simulink model "npc_controller"  (R2022a)
settings: Solver=FixedStepDiscrete  StartTime=0.0  StopTime=20  RelTol=1e-3  EnableMultiTasking=on
values from neighbouring files (symbols this model uses):
  Tsw = 1.5E-5    [param.sldd]
undefined symbols (not defined in the file or in its folder): CAN_O_INT, CANA_BASE, Down, GPTRIP1SEL, GPTRIP2SEL, GPTRIP3SEL, TZ1, TZ2, TZ3, Up
libraries: simulink x153, hdlsllib x90, c2802xlib x34, c2837xDlib x18, c280xlib x12, canmsglib x9, c2838xlib x8, idelinklib_common x3, c2806xlib x2, slpidlib x2, c28004xlib x2, c281xlib x2
(part 38 of 45)

== system npc_controller/CONTROL/STATE-MACHINE/CPU_CONTROL_750_A2_precharge_pfc_ok2_OL SS2/updateSequencePhB/pol_vxn1/neg/SR ON ==
  note: Note:
      | AQCSFRC
      | 0b00 - disables forced PWM
      | 0b01 - forces PWM to LOW
      | 0b10 - forces PWM to  HIGH
  note: Note:A2
      |
      | Function PWM # GPIO # LAUNCHPAD PIN #
      |
      | Synci EPWM1A GPIO0 J4.40
      | EPWM1B GPIO1 J4.39
      |
      | ORPS EPMW6A GPIO10 J8.76
      | EPWM6B GPIO11 J8.75
      |
      | RELAY EPWM3A GPIO4 J4.36
      |
      | TZ GPIO62 XX
      |
      | a_s1 EPWM2A GPIO2 J4.38 XBAR_TRIP4
      | a_s2 EPWM7B GPIO13 XX
      | a_s3 EPWM2B GPIO3 J4.37
      | a_s4 EPWM7A GPIO12 XX XBAR_TRIP5
      |
      | b_s1 EPWM8B GPIO15 J8.73 XBAR_TRIP7
      | b_s2 EPWM9B GPIO17 XX
      | b_s3 EPWM8A GPIO14 J8.74
      | b_s4 EPWM9A GPIO16 J4.33 XBAR_TRIP8
      |
      | c_s1 EPWM10B GPIO19 J1.3 XBAR_TRIP9
      | c_s2 EPWM11B GPIO21 XX
      | c_s3 EPWM10A GPIO18 J1.4
      | c_s4 EPWM11A GPIO20 XX XBAR_TRIP10
  note: EPwm8Regs.AQCSFRC.bit.CSFB = (uint16_T)(0b01);
      | EPwm9Regs.AQCSFRC.bit.CSFB = (uint16_T)(0b00);
      | EPwm8Regs.AQCSFRC.bit.CSFA = (uint16_T)(0b10);
      | EPwm9Regs.AQCSFRC.bit.CSFA = (uint16_T)(0b00);
  Action Port : ActionPort  ActionPortLabel=else
  Constant : Constant  Value=2  OutDataTypeStr=uint8  SampleTime=-1
  System Outputs1 : Subsystem  mask(System Outputs){ShowInLibBrowser=0}
      mask prompts: ShowInLibBrowser "Simulink:masks:CustCodeMaskParam1_MP"
      settings: CopyFcn=cccopyfcn(gcb)  OpenFcn=ccopenfcn('System Outputs Function')
      mask Help: eval('feval(''rtwprivate'',''rtwhelpview'',''rtw_sys_outputs_block'')');
      mask Display: disp('System\nOutputs');
  Out1 : Outport
  wires:
  Constant/1 -> Out1/1

== system npc_controller/CONTROL/STATE-MACHINE/CPU_CONTROL_750_A2_precharge_pfc_ok2_OL SS2/updateSequencePhB/pol_vxn1/pos/SR Force to Low ==
  note: Note:A2
      |
      | Function PWM # GPIO # LAUNCHPAD PIN #
      |
      | Synci EPWM1A GPIO0 J4.40
      | EPWM1B GPIO1 J4.39
      |
      | ORPS EPMW6A GPIO10 J8.76
      | EPWM6B GPIO11 J8.75
      |
      | RELAY EPWM3A GPIO4 J4.36
      |
      | TZ GPIO62 XX
      |
      | a_s1 EPWM2A GPIO2 J4.38 XBAR_TRIP4
      | a_s2 EPWM7B GPIO13 XX
      | a_s3 EPWM2B GPIO3 J4.37
      | a_s4 EPWM7A GPIO12 XX XBAR_TRIP5
      |
      | b_s1 EPWM8B GPIO15 J8.73 XBAR_TRIP7
      | b_s2 EPWM9B GPIO17 XX
      | b_s3 EPWM8A GPIO14 J8.74
      | b_s4 EPWM9A GPIO16 J4.33 XBAR_TRIP8
      |
      | c_s1 EPWM10B GPIO19 J1.3 XBAR_TRIP9
      | c_s2 EPWM11B GPIO21 XX
      | c_s3 EPWM10A GPIO18 J1.4
      | c_s4 EPWM11A GPIO20 XX XBAR_TRIP10
  note: Note:
      | AQCSFRC
      | 0b00 - disables forced PWM
      | 0b01 - forces PWM to LOW
      | 0b10 - forces PWM to  HIGH
  note: EPwm8Regs.AQCSFRC.bit.CSFB = (uint16_T)(0b01);
      | EPwm9Regs.AQCSFRC.bit.CSFB = (uint16_T)(0b10);
      | EPwm8Regs.AQCSFRC.bit.CSFA = (uint16_T)(0b00);
      | EPwm9Regs.AQCSFRC.bit.CSFA = (uint16_T)(0b01);
  Action Port : ActionPort  ActionPortLabel="if((u1 > -48)  & (u1 < 48))"
  Constant : Constant  OutDataTypeStr=uint8  SampleTime=-1
  System Outputs2 : Subsystem  mask(System Outputs){ShowInLibBrowser=0}
      mask prompts: ShowInLibBrowser "Simulink:masks:CustCodeMaskParam1_MP"
      settings: CopyFcn=cccopyfcn(gcb)  OpenFcn=ccopenfcn('System Outputs Function')
      mask Help: eval('feval(''rtwprivate'',''rtwhelpview'',''rtw_sys_outputs_block'')');
      mask Display: disp('System\nOutputs');
  Out1 : Outport
  wires:
  Constant/1 -> Out1/1

== system npc_controller/CONTROL/STATE-MACHINE/CPU_CONTROL_750_A2_precharge_pfc_ok2_OL SS2/updateSequencePhB/pol_vxn1/pos/SR ON ==
  note: Note:
      | AQCSFRC
      | 0b00 - disables forced PWM/pass through
      | 0b01 - forces PWM to LOW
      | 0b10 - forces PWM to  HIGH
  note: Note:A2
      |
      | Function PWM # GPIO # LAUNCHPAD PIN #
      |
      | Synci EPWM1A GPIO0 J4.40
      | EPWM1B GPIO1 J4.39
      |
      | ORPS EPMW6A GPIO10 J8.76
      | EPWM6B GPIO11 J8.75
      |
      | RELAY EPWM3A GPIO4 J4.36
      |
      | TZ GPIO62 XX
      |
      | a_s1 EPWM2A GPIO2 J4.38 XBAR_TRIP4
      | a_s2 EPWM7B GPIO13 XX
      | a_s3 EPWM2B GPIO3 J4.37
      | a_s4 EPWM7A GPIO12 XX XBAR_TRIP5
      |
      | b_s1 EPWM8B GPIO15 J8.73 XBAR_TRIP7
      | b_s2 EPWM9B GPIO17 XX
      | b_s3 EPWM8A GPIO14 J8.74
      | b_s4 EPWM9A GPIO16 J4.33 XBAR_TRIP8
      |
      | c_s1 EPWM10B GPIO19 J1.3 XBAR_TRIP9
      | c_s2 EPWM11B GPIO21 XX
      | c_s3 EPWM10A GPIO18 J1.4
      | c_s4 EPWM11A GPIO20 XX XBAR_TRIP10
  note: EPwm8Regs.AQCSFRC.bit.CSFB = (uint16_T)(0b00);
      | EPwm9Regs.AQCSFRC.bit.CSFB = (uint16_T)(0b10);
      | EPwm8Regs.AQCSFRC.bit.CSFA = (uint16_T)(0b00);
      | EPwm9Regs.AQCSFRC.bit.CSFA = (uint16_T)(0b01);
  Action Port : ActionPort  ActionPortLabel=else
  Constant : Constant  OutDataTypeStr=uint8  SampleTime=-1
  System Outputs1 : Subsystem  mask(System Outputs){ShowInLibBrowser=0}
      mask prompts: ShowInLibBrowser "Simulink:masks:CustCodeMaskParam1_MP"
      settings: CopyFcn=cccopyfcn(gcb)  OpenFcn=ccopenfcn('System Outputs Function')
      mask Help: eval('feval(''rtwprivate'',''rtwhelpview'',''rtw_sys_outputs_block'')');
      mask Display: disp('System\nOutputs');
  Out1 : Outport
  wires:
  Constant/1 -> Out1/1

== system npc_controller/CONTROL/STATE-MACHINE/CPU_CONTROL_750_A2_precharge_pfc_ok2_OL SS2/updateSequencePhB/pol_vxn1/zero/System Outputs1 ==

== system npc_controller/CONTROL/STATE-MACHINE/CPU_CONTROL_750_A2_precharge_pfc_ok2_OL SS2/updateSequencePhB/pol_vxn2/neg/System Outputs1 ==

== system npc_controller/CONTROL/STATE-MACHINE/CPU_CONTROL_750_A2_precharge_pfc_ok2_OL SS2/updateSequencePhB/pol_vxn2/neg/System Outputs2 ==

== system npc_controller/CONTROL/STATE-MACHINE/CPU_CONTROL_750_A2_precharge_pfc_ok2_OL SS2/updateSequencePhB/pol_vxn2/pos/System Outputs1 ==

== system npc_controller/CONTROL/STATE-MACHINE/CPU_CONTROL_750_A2_precharge_pfc_ok2_OL SS2/updateSequencePhB/pol_vxn2/pos/System Outputs2 ==

== system npc_controller/CONTROL/STATE-MACHINE/CPU_CONTROL_750_A2_precharge_pfc_ok2_OL SS2/updateSequencePhB/pol_vxn2/zero/System Outputs1 ==

== system npc_controller/CONTROL/STATE-MACHINE/CPU_CONTROL_750_A2_precharge_pfc_ok2_OL SS2/updateSequencePhC/pol_final1/prot/System Outputs ==

== system npc_controller/CONTROL/STATE-MACHINE/CPU_CONTROL_750_A2_precharge_pfc_ok2_OL SS2/updateSequencePhC/pol_vxn1/neg/SR OFF ==
  note: Note:A2
      |
      | Function PWM # GPIO # LAUNCHPAD PIN #
      |
      | Synci EPWM1A GPIO0 J4.40
      | EPWM1B GPIO1 J4.39
      |
      | ORPS EPMW6A GPIO10 J8.76
      | EPWM6B GPIO11 J8.75
      |
      | RELAY EPWM3A GPIO4 J4.36
      |
      | TZ GPIO62 XX
      |
      | a_s1 EPWM2A GPIO2 J4.38 XBAR_TRIP4
      | a_s2 EPWM7B GPIO13 XX
      | a_s3 EPWM2B GPIO3 J4.37
      | a_s4 EPWM7A GPIO12 XX XBAR_TRIP5
      |
      | b_s1 EPWM8B GPIO15 J8.73 XBAR_TRIP7
      | b_s2 EPWM9B GPIO17 XX
      | b_s3 EPWM8A GPIO14 J8.74
      | b_s4 EPWM9A GPIO16 J4.33 XBAR_TRIP8
      |
      | c_s1 EPWM10B GPIO19 J1.3 XBAR_TRIP9
      | c_s2 EPWM11B GPIO21 XX
      | c_s3 EPWM10A GPIO18 J1.4
      | c_s4 EPWM11A GPIO20 XX XBAR_TRIP10
  note: Note:
      | AQCSFRC
      | 0b00 - disables forced PWM
      | 0b01 - forces PWM to LOW
      | 0b10 - forces PWM to  HIGH
  note: EPwm10Regs.AQCSFRC.bit.CSFB = (uint16_T)(0b01);
      | EPwm11Regs.AQCSFRC.bit.CSFB = (uint16_T)(0b00);
      | EPwm10Regs.AQCSFRC.bit.CSFA = (uint16_T)(0b10);
      | EPwm11Regs.AQCSFRC.bit.CSFA = (uint16_T)(0b01);
  Action Port : ActionPort  ActionPortLabel="if((u1 > -48)  & (u1 < 48))"
  Constant : Constant  Value=2  OutDataTypeStr=uint8  SampleTime=-1
  System Outputs1 : Subsystem  mask(System Outputs){ShowInLibBrowser=0}
      mask prompts: ShowInLibBrowser "Simulink:masks:CustCodeMaskParam1_MP"
      settings: CopyFcn=cccopyfcn(gcb)  OpenFcn=ccopenfcn('System Outputs Function')
      mask Help: eval('feval(''rtwprivate'',''rtwhelpview'',''rtw_sys_outputs_block'')');
      mask Display: disp('System\nOutputs');
  Out1 : Outport
  wires:
  Constant/1 -> Out1/1

== system npc_controller/CONTROL/STATE-MACHINE/CPU_CONTROL_750_A2_precharge_pfc_ok2_OL SS2/updateSequencePhC/pol_vxn1/neg/SR ON ==
  note: Note:
      | AQCSFRC
      | 0b00 - disables forced PWM
      | 0b01 - forces PWM to LOW
      | 0b10 - forces PWM to  HIGH
  note: Note:A2
      |
      | Function PWM # GPIO # LAUNCHPAD PIN #
      |
      | Synci EPWM1A GPIO0 J4.40
      | EPWM1B GPIO1 J4.39
      |
      | ORPS EPMW6A GPIO10 J8.76
      | EPWM6B GPIO11 J8.75
      |
      | RELAY EPWM3A GPIO4 J4.36
      |
      | TZ GPIO62 XX
      |
      | a_s1 EPWM2A GPIO2 J4.38 XBAR_TRIP4
      | a_s2 EPWM7B GPIO13 XX
      | a_s3 EPWM2B GPIO3 J4.37
      | a_s4 EPWM7A GPIO12 XX XBAR_TRIP5
      |
      | b_s1 EPWM8B GPIO15 J8.73 XBAR_TRIP7
      | b_s2 EPWM9B GPIO17 XX
      | b_s3 EPWM8A GPIO14 J8.74
      | b_s4 EPWM9A GPIO16 J4.33 XBAR_TRIP8
      |
      | c_s1 EPWM10B GPIO19 J1.3 XBAR_TRIP9
      | c_s2 EPWM11B GPIO21 XX
      | c_s3 EPWM10A GPIO18 J1.4
      | c_s4 EPWM11A GPIO20 XX XBAR_TRIP10
  note: EPwm10Regs.AQCSFRC.bit.CSFB = (uint16_T)(0b01);
      | EPwm11Regs.AQCSFRC.bit.CSFB = (uint16_T)(0b00);
      | EPwm10Regs.AQCSFRC.bit.CSFA = (uint16_T)(0b10);
      | EPwm11Regs.AQCSFRC.bit.CSFA = (uint16_T)(0b00);
  Action Port : ActionPort  ActionPortLabel=else
  Constant : Constant  Value=2  OutDataTypeStr=uint8  SampleTime=-1
  System Outputs1 : Subsystem  mask(System Outputs){ShowInLibBrowser=0}
      mask prompts: ShowInLibBrowser "Simulink:masks:CustCodeMaskParam1_MP"
      settings: CopyFcn=cccopyfcn(gcb)  OpenFcn=ccopenfcn('System Outputs Function')
      mask Help: eval('feval(''rtwprivate'',''rtwhelpview'',''rtw_sys_outputs_block'')');
      mask Display: disp('System\nOutputs');
  Out1 : Outport
  wires:
  Constant/1 -> Out1/1

== system npc_controller/CONTROL/STATE-MACHINE/CPU_CONTROL_750_A2_precharge_pfc_ok2_OL SS2/updateSequencePhC/pol_vxn1/pos/SR Force to Low ==
  note: Note:A2
      |
      | Function PWM # GPIO # LAUNCHPAD PIN #
      |
      | Synci EPWM1A GPIO0 J4.40
      | EPWM1B GPIO1 J4.39
      |
      | ORPS EPMW6A GPIO10 J8.76
      | EPWM6B GPIO11 J8.75
      |
      | RELAY EPWM3A GPIO4 J4.36
      |
      | TZ GPIO62 XX
      |
      | a_s1 EPWM2A GPIO2 J4.38 XBAR_TRIP4
      | a_s2 EPWM7B GPIO13 XX
      | a_s3 EPWM2B GPIO3 J4.37
      | a_s4 EPWM7A GPIO12 XX XBAR_TRIP5
      |
      | b_s1 EPWM8B GPIO15 J8.73 XBAR_TRIP7
      | b_s2 EPWM9B GPIO17 XX
      | b_s3 EPWM8A GPIO14 J8.74
      | b_s4 EPWM9A GPIO16 J4.33 XBAR_TRIP8
      |
      | c_s1 EPWM10B GPIO19 J1.3 XBAR_TRIP9
      | c_s2 EPWM11B GPIO21 XX
      | c_s3 EPWM10A GPIO18 J1.4
      | c_s4 EPWM11A GPIO20 XX XBAR_TRIP10
  note: Note:
      | AQCSFRC
      | 0b00 - disables forced PWM
      | 0b01 - forces PWM to LOW
      | 0b10 - forces PWM to  HIGH
  note: EPwm10Regs.AQCSFRC.bit.CSFB = (uint16_T)(0b01);
      | EPwm11Regs.AQCSFRC.bit.CSFB = (uint16_T)(0b10);
      | EPwm10Regs.AQCSFRC.bit.CSFA = (uint16_T)(0b00);
      | EPwm11Regs.AQCSFRC.bit.CSFA = (uint16_T)(0b01);
  Action Port : ActionPort  ActionPortLabel="if((u1 > -48)  & (u1 < 48))"
  Constant : Constant  OutDataTypeStr=uint8  SampleTime=-1
  System Outputs2 : Subsystem  mask(System Outputs){ShowInLibBrowser=0}
      mask prompts: ShowInLibBrowser "Simulink:masks:CustCodeMaskParam1_MP"
      settings: CopyFcn=cccopyfcn(gcb)  OpenFcn=ccopenfcn('System Outputs Function')
      mask Help: eval('feval(''rtwprivate'',''rtwhelpview'',''rtw_sys_outputs_block'')');
      mask Display: disp('System\nOutputs');
  Out1 : Outport
  wires:
  Constant/1 -> Out1/1

== system npc_controller/CONTROL/STATE-MACHINE/CPU_CONTROL_750_A2_precharge_pfc_ok2_OL SS2/updateSequencePhC/pol_vxn1/pos/SR ON ==
  note: Note:
      | AQCSFRC
      | 0b00 - disables forced PWM/pass through
      | 0b01 - forces PWM to LOW
      | 0b10 - forces PWM to  HIGH
  note: Note:A2
      |
      | Function PWM # GPIO # LAUNCHPAD PIN #
      |
      | Synci EPWM1A GPIO0 J4.40
      | EPWM1B GPIO1 J4.39
      |
      | ORPS EPMW6A GPIO10 J8.76
      | EPWM6B GPIO11 J8.75
      |
      | RELAY EPWM3A GPIO4 J4.36
      |
      | TZ GPIO62 XX
      |
      | a_s1 EPWM2A GPIO2 J4.38 XBAR_TRIP4
      | a_s2 EPWM7B GPIO13 XX
      | a_s3 EPWM2B GPIO3 J4.37
      | a_s4 EPWM7A GPIO12 XX XBAR_TRIP5
      |
      | b_s1 EPWM8B GPIO15 J8.73 XBAR_TRIP7
      | b_s2 EPWM9B GPIO17 XX
      | b_s3 EPWM8A GPIO14 J8.74
      | b_s4 EPWM9A GPIO16 J4.33 XBAR_TRIP8
      |
      | c_s1 EPWM10B GPIO19 J1.3 XBAR_TRIP9
      | c_s2 EPWM11B GPIO21 XX
      | c_s3 EPWM10A GPIO18 J1.4
      | c_s4 EPWM11A GPIO20 XX XBAR_TRIP10
  note: EPwm10Regs.AQCSFRC.bit.CSFB = (uint16_T)(0b00);
      | EPwm11Regs.AQCSFRC.bit.CSFB = (uint16_T)(0b10);
      | EPwm10Regs.AQCSFRC.bit.CSFA = (uint16_T)(0b00);
      | EPwm11Regs.AQCSFRC.bit.CSFA = (uint16_T)(0b01);
  Action Port : ActionPort  ActionPortLabel=else
  Constant : Constant  OutDataTypeStr=uint8  SampleTime=-1
  System Outputs1 : Subsystem  mask(System Outputs){ShowInLibBrowser=0}
      mask prompts: ShowInLibBrowser "Simulink:masks:CustCodeMaskParam1_MP"
      settings: CopyFcn=cccopyfcn(gcb)  OpenFcn=ccopenfcn('System Outputs Function')
      mask Help: eval('feval(''rtwprivate'',''rtwhelpview'',''rtw_sys_outputs_block'')');
      mask Display: disp('System\nOutputs');
  Out1 : Outport
  wires:
  Constant/1 -> Out1/1

== system npc_controller/CONTROL/STATE-MACHINE/CPU_CONTROL_750_A2_precharge_pfc_ok2_OL SS2/updateSequencePhC/pol_vxn1/zero/System Outputs1 ==

== system npc_controller/CONTROL/STATE-MACHINE/CPU_CONTROL_750_A2_precharge_pfc_ok2_OL SS2/updateSequencePhC/pol_vxn2/neg/System Outputs1 ==

== system npc_controller/CONTROL/STATE-MACHINE/CPU_CONTROL_750_A2_precharge_pfc_ok2_OL SS2/updateSequencePhC/pol_vxn2/pos/System Outputs1 ==

== system npc_controller/CONTROL/STATE-MACHINE/CPU_CONTROL_750_A2_precharge_pfc_ok2_OL SS2/updateSequencePhC/pol_vxn2/pos/System Outputs2 ==

== system npc_controller/CONTROL/STATE-MACHINE/CPU_CONTROL_750_A2_precharge_pfc_ok2_OL SS2/updateSequencePhC/pol_vxn2/zero/System Outputs1 ==

== system npc_controller/CONTROL/STATE-MACHINE/CPU_CONTROL_750_Vpk/configGrid/FORCE_TZ/1P/ALL_LEGS ==
  note: Note:
      | TZCCTL
      | 0b00 - High impedance
      | 0b01 - Force to HIGH
      | 0b10 - Force to LOW
      | 0b11 - Do nothing
      |
      | AQCSFRC
      | 0b00 - disables forced PWM
      | 0b01 - forces PWM to LOW
      | 0b10 - forces PWM to  HIGH
      |
      | TZFRC.bit.OST
      | 0b0 - Do nothing
      | 0b1 - Force TZ
  note: EALLOW;
      |
      | /*Force TZ*/
      | EPwm6Regs. TZFRC.bit.OST = 0b0; //do nothing
      | EPwm7Regs. TZFRC.bit.OST = 0b0;
      | EPwm8Regs. TZFRC.bit.OST = 0b0;
      | EPwm9Regs. TZFRC.bit.OST = 0b0;
      | EPwm10Regs. TZFRC.bit.OST = 0b0;
      | EPwm11Regs. TZFRC.bit.OST = 0b0;
      |
      | EDIS;
      |
      | //change ref for leg B and legC
  Action Port : ActionPort
  System Outputs2 : Subsystem  mask(System Outputs){ShowInLibBrowser=0}
      mask prompts: ShowInLibBrowser "Simulink:masks:CustCodeMaskParam1_MP"
      settings: CopyFcn=cccopyfcn(gcb)  OpenFcn=ccopenfcn('System Outputs Function')
      mask Help: eval('feval(''rtwprivate'',''rtwhelpview'',''rtw_sys_outputs_block'')');
      mask Display: disp('System\nOutputs');

== system npc_controller/CONTROL/STATE-MACHINE/CPU_CONTROL_750_Vpk/configGrid/FORCE_TZ/1P/LEG_A ==
  note: EALLOW;
      |
      | /*Force TZ*/
      | EPwm6Regs. TZFRC.bit.OST = 0b0; //do nothing
      | EPwm7Regs. TZFRC.bit.OST = 0b0;
      | EPwm8Regs. TZFRC.bit.OST = 0b1;
      | EPwm9Regs. TZFRC.bit.OST = 0b1;
      | EPwm10Regs. TZFRC.bit.OST = 0b1;
      | EPwm11Regs. TZFRC.bit.OST = 0b1;
      |
      | EDIS;
  note: Note:
      | TZCCTL
      | 0b00 - High impedance
      | 0b01 - Force to HIGH
      | 0b10 - Force to LOW
      | 0b11 - Do nothing
      |
      | AQCSFRC
      | 0b00 - disables forced PWM
      | 0b01 - forces PWM to LOW
      | 0b10 - forces PWM to  HIGH
      |
      | TZFRC.bit.OST
      | 0b0 - Do nothing
      | 0b1 - Force TZ
  Action Port : ActionPort
  System Outputs2 : Subsystem  mask(System Outputs){ShowInLibBrowser=0}
      mask prompts: ShowInLibBrowser "Simulink:masks:CustCodeMaskParam1_MP"
      settings: CopyFcn=cccopyfcn(gcb)  OpenFcn=ccopenfcn('System Outputs Function')
      mask Help: eval('feval(''rtwprivate'',''rtwhelpview'',''rtw_sys_outputs_block'')');
      mask Display: disp('System\nOutputs');

== system npc_controller/CONTROL/STATE-MACHINE/CPU_CONTROL_750_Vpk/configGrid/FORCE_TZ/1P/LEG_B ==
  note: Note:
      | TZCCTL
      | 0b00 - High impedance
      | 0b01 - Force to HIGH
      | 0b10 - Force to LOW
      | 0b11 - Do nothing
      |
      | AQCSFRC
      | 0b00 - disables forced PWM
      | 0b01 - forces PWM to LOW
      | 0b10 - forces PWM to  HIGH
      |
      | TZFRC.bit.OST
      | 0b0 - Do nothing
      | 0b1 - Force TZ
  note: EALLOW;
      |
      | /*Force TZ*/
      | EPwm6Regs. TZFRC.bit.OST = 0b1; //do nothing
      | EPwm7Regs. TZFRC.bit.OST = 0b1;
      | EPwm8Regs. TZFRC.bit.OST = 0b0;
      | EPwm9Regs. TZFRC.bit.OST = 0b0;
      | EPwm10Regs. TZFRC.bit.OST = 0b1;
      | EPwm11Regs. TZFRC.bit.OST = 0b1;
      |
      | EDIS;
  Action Port : ActionPort
  System Outputs2 : Subsystem  mask(System Outputs){ShowInLibBrowser=0}
      mask prompts: ShowInLibBrowser "Simulink:masks:CustCodeMaskParam1_MP"
      settings: CopyFcn=cccopyfcn(gcb)  OpenFcn=ccopenfcn('System Outputs Function')
      mask Help: eval('feval(''rtwprivate'',''rtwhelpview'',''rtw_sys_outputs_block'')');
      mask Display: disp('System\nOutputs');

== system npc_controller/CONTROL/STATE-MACHINE/CPU_CONTROL_750_Vpk/configGrid/FORCE_TZ/1P/LEG_C ==
  note: EALLOW;
      |
      | /*Force TZ*/
      | EPwm6Regs. TZFRC.bit.OST = 0b1; //do nothing
      | EPwm7Regs. TZFRC.bit.OST = 0b1;
      | EPwm8Regs. TZFRC.bit.OST = 0b1;
      | EPwm9Regs. TZFRC.bit.OST = 0b1;
      | EPwm10Regs. TZFRC.bit.OST = 0b0;
      | EPwm11Regs. TZFRC.bit.OST = 0b0;
      |
      | EDIS;
  note: Note:
      | TZCCTL
      | 0b00 - High impedance
      | 0b01 - Force to HIGH
      | 0b10 - Force to LOW
      | 0b11 - Do nothing
      |
      | AQCSFRC
      | 0b00 - disables forced PWM
      | 0b01 - forces PWM to LOW
      | 0b10 - forces PWM to  HIGH
      |
      | TZFRC.bit.OST
      | 0b0 - Do nothing
      | 0b1 - Force TZ
  Action Port : ActionPort
  System Outputs2 : Subsystem  mask(System Outputs){ShowInLibBrowser=0}
      mask prompts: ShowInLibBrowser "Simulink:masks:CustCodeMaskParam1_MP"
      settings: CopyFcn=cccopyfcn(gcb)  OpenFcn=ccopenfcn('System Outputs Function')
      mask Help: eval('feval(''rtwprivate'',''rtwhelpview'',''rtw_sys_outputs_block'')');
      mask Display: disp('System\nOutputs');

== system npc_controller/CONTROL/STATE-MACHINE/CPU_CONTROL_750_Vpk/configGrid/FORCE_TZ/3P3W/System Outputs2 ==

== system npc_controller/CONTROL/STATE-MACHINE/CPU_CONTROL_750_Vpk/updateCalib/done/RESET_TZ/System Outputs2 ==

== system npc_controller/CONTROL/STATE-MACHINE/CPU_CONTROL_750_Vpk/updatePll3p/PLL/SRF_PLL/Integrator ==
  PI Out : Inport  OutDataTypeStr=single
  Accumulation : Subsystem  TreatAsAtomicUnit=on
  Add : Sum  AccumDataTypeStr=single
  Compare To Constant : simulink/Logic and Bit Operations/Compare To Constant  relop=>=  const=2*pi  OutDataTypeStr=boolean
  If : If  IfExpression=u1
  Merge : Merge
  Product : Product  OutDataTypeStr=single
  Reset Integrator : Subsystem  TreatAsAtomicUnit=on
  Ts : Constant  Value=Tsw  OutDataTypeStr=single
  Unit Delay : UnitDelay  SampleTime=-1  HasFrameUpgradeWarning=on
  wt : Outport
  wires:
  PI Out/1 -> Product/1
  Ts/1 -> Product/2
  Product/1 -> Add/1
  Add/1 -> Accumulation/1(In1), Compare To Constant/1
  Compare To Constant/1 -> If/1
  If/1 -> Reset Integrator/Action
  If/2 -> Accumulation/Action
  Reset Integrator/1(Out) -> Merge/1
  Accumulation/1(Out) -> Merge/2
  Merge/1 -> Unit Delay/1
  Unit Delay/1 -> wt/1, Add/2

== system npc_controller/CONTROL/STATE-MACHINE/CPU_CONTROL_750_Vpk/updatePll3p/PLL/SRF_PLL/PI ==
  Vq : Inport
  Ki : Gain  Gain=200
  Ki1 : Gain  Commented=on  Gain=200
  Kp : Gain  Gain=0.5
  Kp1 : Gain  Commented=on  Gain=0.5
  Sum : Sum  Inputs=|++
  Sum1 : Sum  Inputs=+|+
  Ts/2 : Gain  Gain=Tsw/2
  Unit Delay : UnitDelay  SampleTime=-1  HasFrameUpgradeWarning=on
  PI Out : Outport
  wires:
  Ts/2/1 -> Sum/1
  Sum1/1 -> PI Out/1
  Ki/1 -> Ts/2/1
  Vq/1 -> Ki/1, Kp/1  "Vq"
  Unit Delay/1 -> Sum/2
  Kp/1 -> Sum1/1
  Sum/1 -> Sum1/2, Unit Delay/1

== system npc_controller/CONTROL/STATE-MACHINE/CPU_CONTROL_750_Vpk/updatePll3p/PLL/SRF_PLL/Subsystem1 ==
  x[n] : Inport
  1 - Lambda : Gain  Gain=1 - 0.98
  Delay : Delay  DelayLength=1
  Gain{,1..7} (8 alike) : Gain  Commented=on  Gain=1/8
  Lambda : Gain  Gain=0.98
  Memory{,1..6} (7 alike) : Memory  Commented=on  InheritSampleTime=on
  Sum{,1..6} (7 alike) : Sum  Commented=on  Inputs=++|
  Sum7 : Sum  Inputs=|++
  y[n] : Outport
  wires:
  Sum7/1 -> y[n]/1, Delay/1
  Delay/1 -> Lambda/1
  1 - Lambda/1 -> Sum7/1
  x[n]/1 -> 1 - Lambda/1
  Lambda/1 -> Sum7/2
  Gain7/1 -> Sum6/1
  Sum5/1 -> Sum6/2
  Memory6/1 -> Gain7/1
  Memory5/1 -> Gain6/1, Memory6/1
  Sum4/1 -> Sum5/2
  Gain6/1 -> Sum5/1
  Gain5/1 -> Sum4/1
  Sum3/1 -> Sum4/2
  Memory4/1 -> Gain5/1, Memory5/1
  Memory3/1 -> Gain4/1, Memory4/1
  Sum2/1 -> Sum3/2
  Gain4/1 -> Sum3/1
  Gain3/1 -> Sum2/1
  Sum1/1 -> Sum2/2
  Gain2/1 -> Sum1/1
  Sum/1 -> Sum1/2
  Gain1/1 -> Sum/1
  Gain/1 -> Sum/2
  Memory2/1 -> Gain3/1, Memory3/1
  Memory1/1 -> Gain2/1, Memory2/1
  Memory/1 -> Gain1/1, Memory1/1

== system npc_controller/CONTROL/STATE-MACHINE/CPU_CONTROL_750_Vpk/updatePll3p/PLL/SRF_PLL/abc to dq ==
  note: wt
  note: wt
  note: wt
  a : Inport
  b : Inport  Port=2
  c : Inport  Port=3
  wt : Inport  Port=4
  (wt+120) : Sum  Inputs=|++
  (wt-120) : Sum  Inputs=|+-
  2pi_3 : Constant  Value=2*pi/3
  Add3 : Sum  Inputs=+++
  Cos3 : Trigonometry  Operator=cos
  Cos4 : Trigonometry  Operator=cos
  Cos5 : Trigonometry  Operator=cos
  Product5 : Product
  Product6 : Product
  Product7 : Product
  q1 : Gain  Gain=2/3
  q : Outport
  wires:
  [a] -> Product5/1
  Cos3/1 -> Product5/2
  wt/1 -> (wt+120)/1, (wt-120)/1, Cos3/1
  [ph] -> (wt+120)/2
  Product7/1 -> Add3/3
  a/1 -> [a]
  (wt+120)/1 -> Cos5/1
  Product6/1 -> Add3/2
  c/1 -> [c]
  [ph] -> (wt-120)/2
  (wt-120)/1 -> Cos4/1
  [b] -> Product6/1
  Cos4/1 -> Product6/2
  Product5/1 -> Add3/1
  Cos5/1 -> Product7/2
  b/1 -> [b]
  Add3/1 -> q1/1
  [c] -> Product7/1
  q1/1 -> q/1
  2pi_3/1 -> [ph]

== system npc_controller/CONTROL/STATE-MACHINE/CPU_CONTROL_750_Vpk/updatePll3p/PLL/Subsystem/Initialize at Zero Crossing ==
  In1 : Inport
  Trigger : TriggerPort  VariantControl=Variant
  OR : Logic  Operator=OR  IconShape=distinctive  AllPortsSameDT=off  OutDataTypeStr=boolean
  Unit Delay : UnitDelay  SampleTime=-1  HasFrameUpgradeWarning=on
  Out1 : Outport  InitialOutput=0  VectorParamsAs1DForOutWhenUnconnected=off
  wires:
  OR/1 -> Out1/1, Unit Delay/1
  Unit Delay/1 -> OR/2
  In1/1 -> OR/1

== system npc_controller/CONTROL/STATE-MACHINE/CPU_CONTROL_750_Vpk/updateSequencePhA/pol_final1/prot/System Outputs ==

== system npc_controller/CONTROL/STATE-MACHINE/CPU_CONTROL_750_Vpk/updateSequencePhA/pol_vxn1/neg/System Outputs1 ==

== system npc_controller/CONTROL/STATE-MACHINE/CPU_CONTROL_750_Vpk/updateSequencePhA/pol_vxn1/pos/System Outputs1 ==

== system npc_controller/CONTROL/STATE-MACHINE/CPU_CONTROL_750_Vpk/updateSequencePhA/pol_vxn1/pos/System Outputs2 ==

== system npc_controller/CONTROL/STATE-MACHINE/CPU_CONTROL_750_Vpk/updateSequencePhA/pol_vxn1/zero/System Outputs1 ==

== system npc_controller/CONTROL/STATE-MACHINE/CPU_CONTROL_750_Vpk/updateSequencePhB/pol_final1/prot/System Outputs ==

== system npc_controller/CONTROL/STATE-MACHINE/CPU_CONTROL_750_Vpk/updateSequencePhB/pol_vxn1/neg/System Outputs1 ==

== system npc_controller/CONTROL/STATE-MACHINE/CPU_CONTROL_750_Vpk/updateSequencePhB/pol_vxn1/pos/System Outputs1 ==

== system npc_controller/CONTROL/STATE-MACHINE/CPU_CONTROL_750_Vpk/updateSequencePhB/pol_vxn1/zero/System Outputs1 ==

== system npc_controller/CONTROL/STATE-MACHINE/CPU_CONTROL_750_Vpk/updateSequencePhC/pol_final1/prot/System Outputs ==

== system npc_controller/CONTROL/STATE-MACHINE/CPU_CONTROL_750_Vpk/updateSequencePhC/pol_vxn1/neg/System Outputs1 ==

== system npc_controller/CONTROL/STATE-MACHINE/CPU_CONTROL_750_Vpk/updateSequencePhC/pol_vxn1/pos/System Outputs1 ==

== system npc_controller/CONTROL/STATE-MACHINE/CPU_CONTROL_750_Vpk/updateSequencePhC/pol_vxn1/zero/System Outputs1 ==

== system npc_controller/CONTROL/STATE-MACHINE/CPU_CONTROL_750_precharge_pfc_ok2/configGrid/FORCE_TZ/1P/ALL_LEGS ==
  note: EALLOW;
      |
      | /*Force TZ*/
      | EPwm6Regs. TZFRC.bit.OST = 0b0; //do nothing
      | EPwm7Regs. TZFRC.bit.OST = 0b0;
      | EPwm8Regs. TZFRC.bit.OST = 0b0;
      | EPwm9Regs. TZFRC.bit.OST = 0b0;
      | EPwm10Regs. TZFRC.bit.OST = 0b0;
      | EPwm11Regs. TZFRC.bit.OST = 0b0;
      |
      | EDIS;
      |
      | //change ref for leg B and legC
  note: Note:
      | TZCCTL
      | 0b00 - High impedance
      | 0b01 - Force to HIGH
      | 0b10 - Force to LOW
      | 0b11 - Do nothing
      |
      | AQCSFRC
      | 0b00 - disables forced PWM
      | 0b01 - forces PWM to LOW
      | 0b10 - forces PWM to  HIGH
      |
      | TZFRC.bit.OST
      | 0b0 - Do nothing
      | 0b1 - Force TZ
  Action Port : ActionPort
  System Outputs2 : Subsystem  mask(System Outputs){ShowInLibBrowser=0}
      mask prompts: ShowInLibBrowser "Simulink:masks:CustCodeMaskParam1_MP"
      settings: CopyFcn=cccopyfcn(gcb)  OpenFcn=ccopenfcn('System Outputs Function')
      mask Help: eval('feval(''rtwprivate'',''rtwhelpview'',''rtw_sys_outputs_block'')');
      mask Display: disp('System\nOutputs');

== system npc_controller/CONTROL/STATE-MACHINE/CPU_CONTROL_750_precharge_pfc_ok2/configGrid/FORCE_TZ/1P/LEG_A ==
  note: Note:
      | TZCCTL
      | 0b00 - High impedance
      | 0b01 - Force to HIGH
      | 0b10 - Force to LOW
      | 0b11 - Do nothing
      |
      | AQCSFRC
      | 0b00 - disables forced PWM
      | 0b01 - forces PWM to LOW
      | 0b10 - forces PWM to  HIGH
      |
      | TZFRC.bit.OST
      | 0b0 - Do nothing
      | 0b1 - Force TZ
  note: EALLOW;
      |
      | /*Force TZ*/
      | EPwm6Regs. TZFRC.bit.OST = 0b0; //do nothing
      | EPwm7Regs. TZFRC.bit.OST = 0b0;
      | EPwm8Regs. TZFRC.bit.OST = 0b1;
      | EPwm9Regs. TZFRC.bit.OST = 0b1;
      | EPwm10Regs. TZFRC.bit.OST = 0b1;
      | EPwm11Regs. TZFRC.bit.OST = 0b1;
      |
      | EDIS;
  Action Port : ActionPort
  System Outputs2 : Subsystem  mask(System Outputs){ShowInLibBrowser=0}
      mask prompts: ShowInLibBrowser "Simulink:masks:CustCodeMaskParam1_MP"
      settings: CopyFcn=cccopyfcn(gcb)  OpenFcn=ccopenfcn('System Outputs Function')
      mask Help: eval('feval(''rtwprivate'',''rtwhelpview'',''rtw_sys_outputs_block'')');
      mask Display: disp('System\nOutputs');

== system npc_controller/CONTROL/STATE-MACHINE/CPU_CONTROL_750_precharge_pfc_ok2/configGrid/FORCE_TZ/1P/LEG_B ==
  note: EALLOW;
      |
      | /*Force TZ*/
      | EPwm6Regs. TZFRC.bit.OST = 0b1; //do nothing
      | EPwm7Regs. TZFRC.bit.OST = 0b1;
      | EPwm8Regs. TZFRC.bit.OST = 0b0;
      | EPwm9Regs. TZFRC.bit.OST = 0b0;
      | EPwm10Regs. TZFRC.bit.OST = 0b1;
      | EPwm11Regs. TZFRC.bit.OST = 0b1;
      |
      | EDIS;
  note: Note:
      | TZCCTL
      | 0b00 - High impedance
      | 0b01 - Force to HIGH
      | 0b10 - Force to LOW
      | 0b11 - Do nothing
      |
      | AQCSFRC
      | 0b00 - disables forced PWM
      | 0b01 - forces PWM to LOW
      | 0b10 - forces PWM to  HIGH
      |
      | TZFRC.bit.OST
      | 0b0 - Do nothing
      | 0b1 - Force TZ
  Action Port : ActionPort
  System Outputs2 : Subsystem  mask(System Outputs){ShowInLibBrowser=0}
      mask prompts: ShowInLibBrowser "Simulink:masks:CustCodeMaskParam1_MP"
      settings: CopyFcn=cccopyfcn(gcb)  OpenFcn=ccopenfcn('System Outputs Function')
      mask Help: eval('feval(''rtwprivate'',''rtwhelpview'',''rtw_sys_outputs_block'')');
      mask Display: disp('System\nOutputs');

== system npc_controller/CONTROL/STATE-MACHINE/CPU_CONTROL_750_precharge_pfc_ok2/configGrid/FORCE_TZ/1P/LEG_C ==
  note: Note:
      | TZCCTL
      | 0b00 - High impedance
      | 0b01 - Force to HIGH
      | 0b10 - Force to LOW
      | 0b11 - Do nothing
      |
      | AQCSFRC
      | 0b00 - disables forced PWM
      | 0b01 - forces PWM to LOW
      | 0b10 - forces PWM to  HIGH
      |
      | TZFRC.bit.OST
      | 0b0 - Do nothing
      | 0b1 - Force TZ
  note: EALLOW;
      |
      | /*Force TZ*/
      | EPwm6Regs. TZFRC.bit.OST = 0b1; //do nothing
      | EPwm7Regs. TZFRC.bit.OST = 0b1;
      | EPwm8Regs. TZFRC.bit.OST = 0b1;
      | EPwm9Regs. TZFRC.bit.OST = 0b1;
      | EPwm10Regs. TZFRC.bit.OST = 0b0;
      | EPwm11Regs. TZFRC.bit.OST = 0b0;
      |
      | EDIS;
  Action Port : ActionPort
  System Outputs2 : Subsystem  mask(System Outputs){ShowInLibBrowser=0}
      mask prompts: ShowInLibBrowser "Simulink:masks:CustCodeMaskParam1_MP"
      settings: CopyFcn=cccopyfcn(gcb)  OpenFcn=ccopenfcn('System Outputs Function')
      mask Help: eval('feval(''rtwprivate'',''rtwhelpview'',''rtw_sys_outputs_block'')');
      mask Display: disp('System\nOutputs');

== system npc_controller/CONTROL/STATE-MACHINE/CPU_CONTROL_750_precharge_pfc_ok2/configGrid/FORCE_TZ/3P3W/System Outputs2 ==

== system npc_controller/CONTROL/STATE-MACHINE/CPU_CONTROL_750_precharge_pfc_ok2/updateCalib/done/RESET_TZ/System Outputs2 ==

== system npc_controller/CONTROL/STATE-MACHINE/CPU_CONTROL_750_precharge_pfc_ok2/updatePll3p/PLL/SRF_PLL/Integrator ==
  PI Out : Inport  OutDataTypeStr=single
  Accumulation : Subsystem  TreatAsAtomicUnit=on
  Add : Sum  AccumDataTypeStr=single
  Compare To Constant : simulink/Logic and Bit Operations/Compare To Constant  relop=>=  const=2*pi  OutDataTypeStr=boolean
  If : If  IfExpression=u1
  Merge : Merge
  Product : Product  OutDataTypeStr=single
  Reset Integrator : Subsystem  TreatAsAtomicUnit=on
  Ts : Constant  Value=Tsw  OutDataTypeStr=single
  Unit Delay : UnitDelay  SampleTime=-1  HasFrameUpgradeWarning=on
  wt : Outport
  wires:
  Unit Delay/1 -> Add/2, wt/1
  Merge/1 -> Unit Delay/1
  Accumulation/1(Out) -> Merge/2
  Reset Integrator/1(Out) -> Merge/1
  If/2 -> Accumulation/Action
  If/1 -> Reset Integrator/Action
  Compare To Constant/1 -> If/1
  Add/1 -> Compare To Constant/1, Accumulation/1(In1)
  Product/1 -> Add/1
  Ts/1 -> Product/2
  PI Out/1 -> Product/1

== system npc_controller/CONTROL/STATE-MACHINE/CPU_CONTROL_750_precharge_pfc_ok2/updatePll3p/PLL/SRF_PLL/PI ==
  Vq : Inport
  Ki : Gain  Gain=200
  Ki1 : Gain  Commented=on  Gain=200
  Kp : Gain  Gain=0.5
  Kp1 : Gain  Commented=on  Gain=0.5
  Sum : Sum  Inputs=|++
  Sum1 : Sum  Inputs=+|+
  Ts/2 : Gain  Gain=Tsw/2
  Unit Delay : UnitDelay  SampleTime=-1  HasFrameUpgradeWarning=on
  PI Out : Outport
  wires:
  Sum/1 -> Unit Delay/1, Sum1/2
  Kp/1 -> Sum1/1
  Unit Delay/1 -> Sum/2
  Vq/1 -> Kp/1, Ki/1  "Vq"
  Ki/1 -> Ts/2/1
  Sum1/1 -> PI Out/1
  Ts/2/1 -> Sum/1

== system npc_controller/CONTROL/STATE-MACHINE/CPU_CONTROL_750_precharge_pfc_ok2/updatePll3p/PLL/SRF_PLL/Subsystem1 ==
  x[n] : Inport
  1 - Lambda : Gain  Gain=1 - 0.98
  Delay : Delay  DelayLength=1
  Gain{,1..7} (8 alike) : Gain  Commented=on  Gain=1/8
  Lambda : Gain  Gain=0.98
  Memory{,1..6} (7 alike) : Memory  Commented=on  InheritSampleTime=on
  Sum{,1..6} (7 alike) : Sum  Commented=on  Inputs=++|
  Sum7 : Sum  Inputs=|++
  y[n] : Outport
  wires:
  Memory/1 -> Memory1/1, Gain1/1
  Memory1/1 -> Memory2/1, Gain2/1
  Memory2/1 -> Memory3/1, Gain3/1
  Gain/1 -> Sum/2
  Gain1/1 -> Sum/1
  Sum/1 -> Sum1/2
  Gain2/1 -> Sum1/1
  Sum1/1 -> Sum2/2
  Gain3/1 -> Sum2/1
  Gain4/1 -> Sum3/1
  Sum2/1 -> Sum3/2
  Memory3/1 -> Memory4/1, Gain4/1
  Memory4/1 -> Memory5/1, Gain5/1
  Sum3/1 -> Sum4/2
  Gain5/1 -> Sum4/1
  Gain6/1 -> Sum5/1
  Sum4/1 -> Sum5/2
  Memory5/1 -> Memory6/1, Gain6/1
  Memory6/1 -> Gain7/1
  Sum5/1 -> Sum6/2
  Gain7/1 -> Sum6/1
  Lambda/1 -> Sum7/2
  x[n]/1 -> 1 - Lambda/1
  1 - Lambda/1 -> Sum7/1
  Delay/1 -> Lambda/1
  Sum7/1 -> Delay/1, y[n]/1

== system npc_controller/CONTROL/STATE-MACHINE/CPU_CONTROL_750_precharge_pfc_ok2/updatePll3p/PLL/SRF_PLL/abc to dq ==
  note: wt
  note: wt
  note: wt
  a : Inport
  b : Inport  Port=2
  c : Inport  Port=3
  wt : Inport  Port=4
  (wt+120) : Sum  Inputs=|++
  (wt-120) : Sum  Inputs=|+-
  2pi_3 : Constant  Value=2*pi/3
  Add3 : Sum  Inputs=+++
  Cos3 : Trigonometry  Operator=cos
  Cos4 : Trigonometry  Operator=cos
  Cos5 : Trigonometry  Operator=cos
  Product5 : Product
  Product6 : Product
  Product7 : Product
  q1 : Gain  Gain=2/3
  q : Outport
  wires:
  2pi_3/1 -> [ph]
  q1/1 -> q/1
  [c] -> Product7/1
  Add3/1 -> q1/1
  b/1 -> [b]
  Cos5/1 -> Product7/2
  Product5/1 -> Add3/1
  Cos4/1 -> Product6/2
  [b] -> Product6/1
  (wt-120)/1 -> Cos4/1
  [ph] -> (wt-120)/2
  c/1 -> [c]
  Product6/1 -> Add3/2
  (wt+120)/1 -> Cos5/1
  a/1 -> [a]
  Product7/1 -> Add3/3
  [ph] -> (wt+120)/2
  wt/1 -> Cos3/1, (wt-120)/1, (wt+120)/1
  Cos3/1 -> Product5/2
  [a] -> Product5/1

== system npc_controller/CONTROL/STATE-MACHINE/CPU_CONTROL_750_precharge_pfc_ok2/updatePll3p/PLL/Subsystem/Initialize at Zero Crossing ==
  In1 : Inport
  Trigger : TriggerPort  VariantControl=Variant
  OR : Logic  Operator=OR  IconShape=distinctive  AllPortsSameDT=off  OutDataTypeStr=boolean
  Unit Delay : UnitDelay  SampleTime=-1  HasFrameUpgradeWarning=on
  Out1 : Outport  InitialOutput=0  VectorParamsAs1DForOutWhenUnconnected=off
  wires:
  In1/1 -> OR/1
  Unit Delay/1 -> OR/2
  OR/1 -> Unit Delay/1, Out1/1

== system npc_controller/CONTROL/STATE-MACHINE/CPU_CONTROL_750_precharge_pfc_ok2/updateSequencePhA/pol_final1/prot/System Outputs ==

== system npc_controller/CONTROL/STATE-MACHINE/CPU_CONTROL_750_precharge_pfc_ok2/updateSequencePhA/pol_vxn1/neg/System Outputs1 ==

== system npc_controller/CONTROL/STATE-MACHINE/CPU_CONTROL_750_precharge_pfc_ok2/updateSequencePhA/pol_vxn1/pos/System Outputs1 ==

== system npc_controller/CONTROL/STATE-MACHINE/CPU_CONTROL_750_precharge_pfc_ok2/updateSequencePhA/pol_vxn1/pos/System Outputs2 ==

== system npc_controller/CONTROL/STATE-MACHINE/CPU_CONTROL_750_precharge_pfc_ok2/updateSequencePhA/pol_vxn1/zero/System Outputs1 ==

== system npc_controller/CONTROL/STATE-MACHINE/CPU_CONTROL_750_precharge_pfc_ok2/updateSequencePhB/pol_final1/prot/System Outputs ==

== system npc_controller/CONTROL/STATE-MACHINE/CPU_CONTROL_750_precharge_pfc_ok2/updateSequencePhB/pol_vxn1/neg/System Outputs1 ==

== system npc_controller/CONTROL/STATE-MACHINE/CPU_CONTROL_750_precharge_pfc_ok2/updateSequencePhB/pol_vxn1/pos/System Outputs1 ==

== system npc_controller/CONTROL/STATE-MACHINE/CPU_CONTROL_750_precharge_pfc_ok2/updateSequencePhB/pol_vxn1/zero/System Outputs1 ==

== system npc_controller/CONTROL/STATE-MACHINE/CPU_CONTROL_750_precharge_pfc_ok2/updateSequencePhC/pol_final1/prot/System Outputs ==

== system npc_controller/CONTROL/STATE-MACHINE/CPU_CONTROL_750_precharge_pfc_ok2/updateSequencePhC/pol_vxn1/neg/System Outputs1 ==

== system npc_controller/CONTROL/STATE-MACHINE/CPU_CONTROL_750_precharge_pfc_ok2/updateSequencePhC/pol_vxn1/pos/System Outputs1 ==

== system npc_controller/CONTROL/STATE-MACHINE/CPU_CONTROL_750_precharge_pfc_ok2/updateSequencePhC/pol_vxn1/zero/System Outputs1 ==

== system npc_controller/CONTROL/SVPWM/PLL_Block/SRF_PLL/Integrator/Accumulation ==
  In1 : Inport  OutDataTypeStr=single
  Action Port : ActionPort
  Out : Outport  OutDataTypeStr=single
  wires:
  In1/1 -> Out/1

== system npc_controller/CONTROL/SVPWM/PLL_Block/SRF_PLL/Integrator/Reset Integrator ==
  Action Port : ActionPort
  Constant1 : Constant  Value=0  OutDataTypeStr=single
  Out : Outport
  wires:
  Constant1/1 -> Out/1

== system npc_controller/IDLE_AND_TIMER/codegen/CAN_Task/Rx_Handler/ ProcessMB10/All Legs ==
  Action Port : ActionPort  ActionPortLabel=elseif( u1 == 4)
  Data Store Write1 : DataStoreWrite  DataStoreName=u8SinglePhaseLeg  IndexOptions=Index vector (dialog)  Indices=1  OutputSizes=1
  Leg All : Constant  Value=4  OutDataTypeStr=uint8
  wires:
  Leg All/1 -> Data Store Write1/1

== system npc_controller/IDLE_AND_TIMER/codegen/CAN_Task/Rx_Handler/ ProcessMB10/Leg A ==
  Action Port : ActionPort  ActionPortLabel=if(u1 == 1)
  Data Store Write1 : DataStoreWrite  DataStoreName=u8SinglePhaseLeg  IndexOptions=Index vector (dialog)  Indices=1  OutputSizes=1
  Leg A : Constant  OutDataTypeStr=uint8
  wires:
  Leg A/1 -> Data Store Write1/1

== system npc_controller/IDLE_AND_TIMER/codegen/CAN_Task/Rx_Handler/ ProcessMB10/Leg B ==
  Action Port : ActionPort  ActionPortLabel=elseif(u1 == 2)
  Data Store Write1 : DataStoreWrite  DataStoreName=u8SinglePhaseLeg  IndexOptions=Index vector (dialog)  Indices=1  OutputSizes=1
  Leg B : Constant  Value=2  OutDataTypeStr=uint8
  wires:
  Leg B/1 -> Data Store Write1/1

== system npc_controller/IDLE_AND_TIMER/codegen/CAN_Task/Rx_Handler/ ProcessMB10/Leg C ==
  Action Port : ActionPort  ActionPortLabel=elseif( u1 == 3)
  Data Store Write1 : DataStoreWrite  DataStoreName=u8SinglePhaseLeg  IndexOptions=Index vector (dialog)  Indices=1  OutputSizes=1
  Leg C : Constant  Value=3  OutDataTypeStr=uint8
  wires:
  Leg C/1 -> Data Store Write1/1

== system npc_controller/IDLE_AND_TIMER/codegen/CAN_Task/Rx_Handler/ ProcessMB10/Mode_Cmd ==
  Input : Inport
  Action Port : ActionPort  ActionPortLabel=if(u1 == 1)
  Data Store Write1 : DataStoreWrite  DataStoreName=u8ModeCmd  IndexOptions=Index vector (dialog)  Indices=1  OutputSizes=1
  wires:
  Input/1 -> Data Store Write1/1

== system npc_controller/IDLE_AND_TIMER/codegen/CAN_Task/Rx_Handler/ ProcessMB10/Phase Type 1 Phase ==
  Action Port : ActionPort  ActionPortLabel=if(u1 == 1)
  Data Store Write1 : DataStoreWrite  DataStoreName=u8GridPhaseType  IndexOptions=Index vector (dialog)  Indices=1  OutputSizes=1
  Single Phase : Constant  OutDataTypeStr=uint8
  wires:
  Single Phase/1 -> Data Store Write1/1

== system npc_controller/IDLE_AND_TIMER/codegen/CAN_Task/Rx_Handler/ ProcessMB10/Phase Type 3 Phase ==
  Action Port : ActionPort  ActionPortLabel=else
  Data Store Write1 : DataStoreWrite  DataStoreName=u8GridPhaseType  IndexOptions=Index vector (dialog)  Indices=1  OutputSizes=1
  Three Phase : Constant  Value=0  OutDataTypeStr=uint8
  wires:
  Three Phase/1 -> Data Store Write1/1

== system npc_controller/IDLE_AND_TIMER/codegen/CAN_Task/Rx_Handler/ProcessMB11/Red_Mode_Cmd ==
  Input : Inport
  Action Port : ActionPort  ActionPortLabel=if(u1 == 1)
  Data Store Write1 : DataStoreWrite  DataStoreName=u8RedunModeCmd  IndexOptions=Index vector (dialog)  Indices=1  OutputSizes=1
  wires:
  Input/1 -> Data Store Write1/1

== system npc_controller/IDLE_AND_TIMER/codegen/CAN_Task/Rx_Handler/ProcessMB12/Debug_Cmd ==
  Action Port : ActionPort  ActionPortLabel=elseif( u1==2)
  Constant3 : Constant  Value=[1:1]
  Data Store Read1 : DataStoreRead  DataStoreName=u8CanDataRx12  IndexOptions=Index vector (dialog)  Indices=1  OutputSizes=1
  Debug En/Dis : Subsystem  TreatAsAtomicUnit=on
  FUT En Dis : Subsystem  TreatAsAtomicUnit=on
  If1 : If  IfExpression=u1 == hex2dec('0xDA')  ElseIfExpressions=u1 == hex2dec('0xDB')
  Selector3 : Selector  IndexMode=Zero-based  InputPortWidth=8  IndexOptions=Index vector (port)  Indices=[1 3]  OutputSizes=1
  wires:
  If1/2 -> FUT En Dis/Action
  If1/1 -> Debug En/Dis/Action
  Constant3/1 -> Selector3/2
  Data Store Read1/1 -> Selector3/1
  Selector3/1 -> If1/1

== system npc_controller/IDLE_AND_TIMER/codegen/CAN_Task/Rx_Handler/ProcessMB12/Debug_Read ==
  Action Port : ActionPort  ActionPortLabel=if(u1 == 0)
  Constant2 : Constant  Value=[1:1]
  Data Store Read : DataStoreRead  DataStoreName=u8CanDataRx12  IndexOptions=Index vector (dialog)  Indices=1  OutputSizes=1
  Debug_Cmd : Subsystem  TreatAsAtomicUnit=on
  Equal{,1..3} (4 alike) : RelationalOperator  Operator===  OutDataTypeStr=boolean  RndMeth=Simplest  InputSameDT=off
  If : If  IfExpression=u1 == 1
  OR : Logic  Operator=OR  Inputs=4  IconShape=distinctive  AllPortsSameDT=off  OutDataTypeStr=boolean
  RdReq_Calib : Constant  Value=0xD0
  RdReq_Deb1 : Constant  Value=0xD1
  RdReq_Deb2 : Constant  Value=0xD2
  RdReq_FwRev : Constant  Value=0xF0
  Selector1 : Selector  IndexMode=Zero-based  InputPortWidth=8  IndexOptions=Index vector (port)  Indices=[1 3]  OutputSizes=1
  wires:
  Constant2/1 -> Selector1/2
  Data Store Read/1 -> Selector1/1
  RdReq_FwRev/1 -> Equal/2
  RdReq_Calib/1 -> Equal1/2
  Selector1/1 -> Equal1/1, Equal2/1, Debug_Cmd/1(Input), Equal3/1, Equal/1
  RdReq_Deb2/1 -> Equal3/2
  RdReq_Deb1/1 -> Equal2/2
  Equal2/1 -> OR/3
  Equal3/1 -> OR/4
  Equal1/1 -> OR/2
  Equal/1 -> OR/1
  OR/1 -> If/1
  If/1 -> Debug_Cmd/Action

== system npc_controller/IDLE_AND_TIMER/codegen/CAN_Task/Rx_Handler/ProcessMB12/Debug_Write ==
  Action Port : ActionPort  ActionPortLabel=elseif(u1 ==1)

== system npc_controller/IDLE_AND_TIMER/codegen/CAN_Task/Tx_Handler/Run Tx Routine/TxReadRequest ==
  Action Port : ActionPort  ActionPortLabel=if(u1 == 1 & u2 == 1)
  " Tx FW Rev ID134" : Subsystem  TreatAsAtomicUnit=on
  Constant1 : Constant  Value=0  OutDataTypeStr=boolean
  Data Store Read2 : DataStoreRead  DataStoreName=u8RdReqMsgPntr  IndexOptions=Index vector (dialog)  Indices=1  OutputSizes=1
  Data Store Write1 : DataStoreWrite  DataStoreName=b01_ReadRequest  IndexOptions=Index vector (dialog)  Indices=1  OutputSizes=1
  Switch Case : SwitchCase  CaseConditions={0xF0, 0xD0, 0xD1, 0xD2}  ShowDefaultCase=off
  Tx Cal Data ID135 : Subsystem  TreatAsAtomicUnit=on
  Tx TxDeb Dat1 136 : Subsystem  TreatAsAtomicUnit=on
  Tx TxDeb Dat2 137 : Subsystem  TreatAsAtomicUnit=on
  wires:
  Data Store Read2/1 -> Switch Case/1
  Switch Case/1 -> " Tx FW Rev ID134"/Action
  Switch Case/2 -> Tx Cal Data ID135/Action
  Switch Case/3 -> Tx TxDeb Dat1 136/Action
  Switch Case/4 -> Tx TxDeb Dat2 137/Action
  Constant1/1 -> Data Store Write1/1

== system npc_controller/IDLE_AND_TIMER/codegen/CAN_Task/Tx_Handler/Run Tx Routine/TxStatusData ==
  Action Port : ActionPort  ActionPortLabel=else
  Data Store Read2 : DataStoreRead  DataStoreName=u8CanTxIndex  IndexOptions=Index vector (dialog)  Indices=1  OutputSizes=1
  Switch Case : SwitchCase  CaseConditions={0, 1, 2, 3, 4}  ShowDefaultCase=off
  Tx Pri Status ID110 : Subsystem  TreatAsAtomicUnit=on
  Tx Pri1 ID130 : Subsystem  TreatAsAtomicUnit=on
  Tx Pri2 ID131 : Subsystem  TreatAsAtomicUnit=on
  Tx Pri3 ID132 : Subsystem  TreatAsAtomicUnit=on
  Tx Pri4 ID133 : Subsystem  TreatAsAtomicUnit=on
  wires:
  Data Store Read2/1 -> Switch Case/1
  Switch Case/1 -> Tx Pri Status ID110/Action
  Switch Case/2 -> Tx Pri1 ID130/Action
  Switch Case/3 -> Tx Pri2 ID131/Action
  Switch Case/4 -> Tx Pri3 ID132/Action
  Switch Case/5 -> Tx Pri4 ID133/Action

== system npc_controller/IDLE_AND_TIMER/codegen/IDLE/idle_task/get_adc_tmp_mux/get_tmp_mux_inlet ==
  In1 : Inport
  Action Port : ActionPort  ActionPortLabel=case [ 3 ]:
  Data Store Write13 : DataStoreWrite  DataStoreName=adc_temp_inlet  IndexOptions=Index vector (dialog)  Indices=1  OutputSizes=1
  wires:
  In1/1 -> Data Store Write13/1

== system npc_controller/IDLE_AND_TIMER/codegen/IDLE/idle_task/get_adc_tmp_mux/get_tmp_mux_npca ==
  In1 : Inport
  Action Port : ActionPort  ActionPortLabel=case [ 0 ]:
  Data Store Write13 : DataStoreWrite  DataStoreName=adc_temp_npca  IndexOptions=Index vector (dialog)  Indices=1  OutputSizes=1
  wires:
  In1/1 -> Data Store Write13/1

== system npc_controller/IDLE_AND_TIMER/codegen/IDLE/idle_task/get_adc_tmp_mux/get_tmp_mux_npcb ==
  In1 : Inport
  Action Port : ActionPort  ActionPortLabel=case [ 1 ]:
  Data Store Write13 : DataStoreWrite  DataStoreName=adc_temp_npcb  IndexOptions=Index vector (dialog)  Indices=1  OutputSizes=1
  wires:
  In1/1 -> Data Store Write13/1

== system npc_controller/IDLE_AND_TIMER/codegen/IDLE/idle_task/get_adc_tmp_mux/get_tmp_mux_npcc ==
  In1 : Inport
  Action Port : ActionPort  ActionPortLabel=case [ 2 ]:
  Data Store Write13 : DataStoreWrite  DataStoreName=adc_temp_npcc  IndexOptions=Index vector (dialog)  Indices=1  OutputSizes=1
  wires:
  In1/1 -> Data Store Write13/1

== system npc_controller/IDLE_AND_TIMER/codegen/IDLE/idle_task/hkeep/tfv ==
  function : TriggerPort  TriggerType=function-call  VariantControl=Variant
  hkeep1 : Stateflow chart  TreatAsAtomicUnit=on

== system npc_controller/IDLE_AND_TIMER/codegen/IDLE/idle_task/hkeep/tz ==
  note: Reading the trip zone flag from epwm2 and writing to tz_ocp and tz_ovp flags
  note: npc_controller_DWork .tz_ocp = EPwm2Regs.TZOSTFLG.bit.OST1;
      | npc_controller_DWork .tz_ovp = EPwm2Regs.TZOSTFLG.bit.OST2;
      |
      | /*npc_controller_DWork .tz_cmpssocp = EPwm2Regs.TZOSTFLG.bit.DCAEVT1 | EPwm2Regs.TZOSTFLG.bit.DCBEVT1 | EPwm7Regs.TZOSTFLG.bit.DCAEVT1 | EPwm7Regs.TZOSTFLG.bit.DCBEVT1 | EPwm8Regs.TZOSTFLG.bit.DCAEVT1 | EPwm8Regs.TZOSTFLG.bit.DCBEVT1 | EPwm9Regs.TZOSTFLG.bit.DCAEVT1 | EPwm9Regs.TZOSTFLG.bit.DCBEVT1| EPwm10Regs.TZOSTFLG.bit.DCAEVT1 | EPwm10Regs.TZOSTFLG.bit.DCBEVT1 | EPwm11Regs.TZOSTFLG.bit.DCAEVT1 | EPwm11Regs.TZOSTFLG.bit.DCBEVT1;*/
      |
      | /*npc_controller_DWork .tz_cmpssocp = EPwm2Regs.TZFLG.bit.DCAEVT1 | EPwm2Regs.TZFLG.bit.DCBEVT1 | EPwm7Regs.TZFLG.bit.DCAEVT1 | EPwm7Regs.TZFLG.bit.DCBEVT1 | EPwm8Regs.TZFLG.bit.DCAEVT1 | EPwm8Regs.TZFLG.bit.DCBEVT1 | EPwm9Regs.TZFLG.bit.DCAEVT1 | EPwm9Regs.TZFLG.bit.DCBEVT1| EPwm10Regs.TZFLG.bit.DCAEVT1 | EPwm10Regs.TZFLG.bit.DCBEVT1 | EPwm11Regs.TZFLG.bit.DCAEVT1 | EPwm11Regs.TZFLG.bit.DCBEVT1;*/
      |
      | /*npc_controller_DWork .tz_ocp = EPwm7Regs.TZOSTFLG.bit.OST1;
      | npc_controller_DWork .tz_ovp = EPwm7Regs.TZOSTFLG.bit.OST2;
      |
      | npc_controller_DWork .tz_ocp = EPwm8Regs.TZOSTFLG.bit.OST1;
      | npc_controller_DWork .tz_ovp = EPwm8Regs.TZOSTFLG.bit.OST2;
      |
      | npc_controller_DWork .tz_ocp = EPwm9Regs.TZOSTFLG.bit.OST1;
      | npc_controller_DWork .tz_ovp = EPwm9Regs.TZOSTFLG.bit.OST2;
      |
      | npc_controller_DWork .tz_ocp = EPwm10Regs.TZOSTFLG.bit.OST1;
      | npc_controller_DWork .tz_ovp = EPwm10Regs.TZOSTFLG.bit.OST2;
      |
      | npc_controller_DWork .tz_ocp = EPwm11Regs.TZOSTFLG.bit.OST1;
      | npc_controller_DWork .tz_ovp = EPwm11Regs.TZOSTFLG.bit.OST2;*/
  function : TriggerPort  TriggerType=function-call  VariantControl=Variant
  System Outputs2 : Subsystem  mask(System Outputs){ShowInLibBrowser=0}
      mask prompts: ShowInLibBrowser "Simulink:masks:CustCodeMaskParam1_MP"
      settings: CopyFcn=cccopyfcn(gcb)  OpenFcn=ccopenfcn('System Outputs Function')
      mask Help: eval('feval(''rtwprivate'',''rtwhelpview'',''rtw_sys_outputs_block'')');
      mask Display: disp('System\nOutputs');

== system npc_controller/IDLE_AND_TIMER/codegen/IDLE/idle_task/hkeep/tz1 ==
  note: npc_controller_DWork .tz_ocp = EPwm2Regs.TZOSTFLG.bit.OST1;
      | npc_controller_DWork .tz_ovp = EPwm2Regs.TZOSTFLG.bit.OST2;
      |
      | /*npc_controller_DWork .tz_ocp = EPwm7Regs.TZOSTFLG.bit.OST1;
      | npc_controller_DWork .tz_ovp = EPwm7Regs.TZOSTFLG.bit.OST2;
      |
      | npc_controller_DWork .tz_ocp = EPwm8Regs.TZOSTFLG.bit.OST1;
      | npc_controller_DWork .tz_ovp = EPwm8Regs.TZOSTFLG.bit.OST2;
      |
      | npc_controller_DWork .tz_ocp = EPwm9Regs.TZOSTFLG.bit.OST1;
      | npc_controller_DWork .tz_ovp = EPwm9Regs.TZOSTFLG.bit.OST2;
      |
      | npc_controller_DWork .tz_ocp = EPwm10Regs.TZOSTFLG.bit.OST1;
      | npc_controller_DWork .tz_ovp = EPwm10Regs.TZOSTFLG.bit.OST2;
      |
      | npc_controller_DWork .tz_ocp = EPwm11Regs.TZOSTFLG.bit.OST1;
      | npc_controller_DWork .tz_ovp = EPwm11Regs.TZOSTFLG.bit.OST2;*/
  note: Reading the trip zone flag from epwm2 and writing to tz_ocp and tz_ovp flags
  function : TriggerPort  TriggerType=function-call  VariantControl=Variant
  System Outputs2 : Subsystem  mask(System Outputs){ShowInLibBrowser=0}
      mask prompts: ShowInLibBrowser "Simulink:masks:CustCodeMaskParam1_MP"
      settings: CopyFcn=cccopyfcn(gcb)  OpenFcn=ccopenfcn('System Outputs Function')
      mask Help: eval('feval(''rtwprivate'',''rtwhelpview'',''rtw_sys_outputs_block'')');
      mask Display: disp('System\nOutputs');

== system npc_controller/IDLE_AND_TIMER/codegen/IDLE/idle_task/report_adc/Subsystem1 ==
  adc : Inport
  zero_offset : Inport  Port=2
  gain : Inport  Port=3
  Product6 : Product  OutDataTypeStr=single
  Saturation : Saturate  UpperLimit=inf  LowerLimit=0
  Subtract : Sum  Inputs=+-  AccumDataTypeStr=single  OutDataTypeStr=single
  actual : Outport
  wires:
  Saturation/1 -> Product6/1
  Subtract/1 -> Saturation/1
  zero_offset/1 -> Subtract/2
  adc/1 -> Subtract/1
  gain/1 -> Product6/2
  Product6/1 -> actual/1

== system npc_controller/IDLE_AND_TIMER/codegen/IDLE/idle_task/report_adc/Subsystem10 ==
  adc : Inport
  gain : Inport  Port=2
  Product6 : Product  OutDataTypeStr=single
  actual : Outport
  wires:
  Product6/1 -> actual/1
  gain/1 -> Product6/2
  adc/1 -> Product6/1

== system npc_controller/IDLE_AND_TIMER/codegen/IDLE/idle_task/report_adc/Subsystem11 ==
  adc : Inport
  zero_offset : Inport  Port=2
  gain : Inport  Port=3
  Product6 : Product  OutDataTypeStr=single
  Saturation : Saturate  UpperLimit=inf  LowerLimit=0
  Subtract : Sum  Inputs=+-  AccumDataTypeStr=single  OutDataTypeStr=single
  actual : Outport
  wires:
  Product6/1 -> actual/1
  gain/1 -> Product6/2
  adc/1 -> Subtract/1
  zero_offset/1 -> Subtract/2
  Subtract/1 -> Saturation/1
  Saturation/1 -> Product6/1

== system npc_controller/IDLE_AND_TIMER/codegen/IDLE/idle_task/report_adc/Subsystem2 ==
  adc : Inport
  zero_offset : Inport  Port=2
  gain : Inport  Port=3
  Product6 : Product  OutDataTypeStr=single
  Saturation : Saturate  UpperLimit=inf  LowerLimit=0
  Subtract : Sum  Inputs=+-  AccumDataTypeStr=single  OutDataTypeStr=single
  actual : Outport
  wires:
  Product6/1 -> actual/1
  gain/1 -> Product6/2
  adc/1 -> Subtract/1
  zero_offset/1 -> Subtract/2
  Subtract/1 -> Saturation/1
  Saturation/1 -> Product6/1

== system npc_controller/IDLE_AND_TIMER/codegen/IDLE/idle_task/report_adc/Subsystem3 ==
  adc : Inport
  zero_offset : Inport  Port=2
  gain : Inport  Port=3
  Product6 : Product  OutDataTypeStr=single
  Saturation : Saturate  UpperLimit=inf  LowerLimit=0
  Subtract : Sum  Inputs=+-  AccumDataTypeStr=single  OutDataTypeStr=single
  actual : Outport
  wires:
  Saturation/1 -> Product6/1
  Subtract/1 -> Saturation/1
  zero_offset/1 -> Subtract/2
  adc/1 -> Subtract/1
  gain/1 -> Product6/2
  Product6/1 -> actual/1

== system npc_controller/IDLE_AND_TIMER/codegen/IDLE/idle_task/report_adc/Subsystem4 ==
  adc : Inport
  zero_offset : Inport  Port=2
  gain : Inport  Port=3
  Product6 : Product  OutDataTypeStr=single
  Saturation : Saturate  UpperLimit=inf  LowerLimit=0
  Subtract : Sum  Inputs=+-  AccumDataTypeStr=single  OutDataTypeStr=single
  actual : Outport
  wires:
  Product6/1 -> actual/1
  gain/1 -> Product6/2
  adc/1 -> Subtract/1
  zero_offset/1 -> Subtract/2
  Subtract/1 -> Saturation/1
  Saturation/1 -> Product6/1

== system npc_controller/IDLE_AND_TIMER/codegen/IDLE/idle_task/report_adc/Subsystem5 ==
  adc : Inport
  zero_offset : Inport  Port=2
  gain : Inport  Port=3
  Product6 : Product  OutDataTypeStr=single
  Saturation : Saturate  UpperLimit=inf  LowerLimit=0
  Subtract : Sum  Inputs=+-  AccumDataTypeStr=single  OutDataTypeStr=single
  actual : Outport
  wires:
  Saturation/1 -> Product6/1
  Subtract/1 -> Saturation/1
  zero_offset/1 -> Subtract/2
  adc/1 -> Subtract/1
  gain/1 -> Product6/2
  Product6/1 -> actual/1

== system npc_controller/IDLE_AND_TIMER/codegen/IDLE/idle_task/report_adc/Subsystem6 ==
  adc : Inport
  zero_offset : Inport  Port=2
  gain : Inport  Port=3
  Product6 : Product  OutDataTypeStr=single
  Saturation : Saturate  UpperLimit=inf  LowerLimit=0
  Subtract : Sum  Inputs=+-  AccumDataTypeStr=single  OutDataTypeStr=single
  actual : Outport
  wires:
  Product6/1 -> actual/1
  gain/1 -> Product6/2
  adc/1 -> Subtract/1
  zero_offset/1 -> Subtract/2
  Subtract/1 -> Saturation/1
  Saturation/1 -> Product6/1

== system npc_controller/IDLE_AND_TIMER/codegen/IDLE/idle_task/report_adc/Subsystem7 ==
  adc : Inport
  zero_offset : Inport  Port=2
  gain : Inport  Port=3
  Product6 : Product  OutDataTypeStr=single
  Saturation : Saturate  UpperLimit=inf  LowerLimit=0
  Subtract : Sum  Inputs=+-  AccumDataTypeStr=single  OutDataTypeStr=single
  actual : Outport
  wires:
  Product6/1 -> actual/1
  gain/1 -> Product6/2
  adc/1 -> Subtract/1
  zero_offset/1 -> Subtract/2
  Subtract/1 -> Saturation/1
  Saturation/1 -> Product6/1
